simulink model "JFK_Sleep_u"  (R2015a)
settings: Solver=ode3  StartTime=0.0  StopTime=3000  FixedStep=0.01  RelTol=1e-5
values from neighbouring files (symbols this model uses):
  D = 1600/24    (= 66.6666666667)    [Periodic_Solution.m]
  H0 = 0.4    [Periodic_Solution.m]
  T = 24    [Periodic_Solution.m]
  umax = 0.1731    [Periodic_Solution.m]
  x0 = 1.06    [Periodic_Solution.m]
  xc0 = 0    [Periodic_Solution.m]
settings Model: Creator=Zhang Jiaxiang  LastModifiedBy=Jiawei Yin
settings DataIOCC: LimitDataPoints=off  SignalLoggingSaveFormat=ModelDataLogs
settings OptimizationCC: ExpressionDepthLimit=2147483647
settings DebuggingCC: UnderspecifiedInitializationDetection=Classic  MergeDetectMultiDrivingBlocksExec=none  FcnCallInpInsideContextMsg=UseLocalSettings  StateNameClashWarn=warning
settings GRTTargetCC: CombineOutputUpdateFcns=off  GRTInterface=on

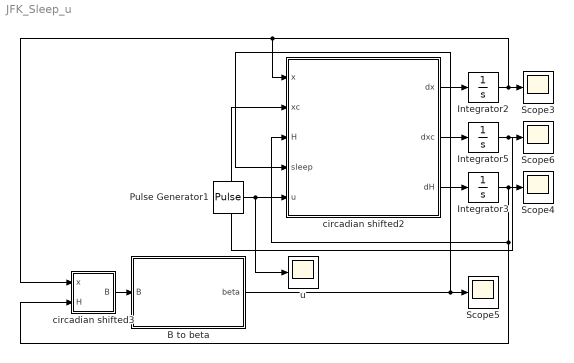
== system JFK_Sleep_u ==
  B to beta : Subsystem
  Integrator2 : Integrator  InitialCondition=x0
  Integrator3 : Integrator  InitialCondition=H0
  Integrator5 : Integrator  InitialCondition=xc0
  Pulse Generator1 : DiscretePulseGenerator  PulseType=Time based  Amplitude=umax  Period=T  PulseWidth=D
  Scope{3..6} (4 alike) : Scope
      Scope3 settings: TimeRange=auto  MaxDataPoints=5000  SaveName=x  YMin=-1.3407  YMax=1.30997  SampleTime=-1  DataFormat=Array
      Scope4 settings: TimeRange=auto  MaxDataPoints=5000  SaveName=H  YMin=0.02024  YMax=0.68165  SampleTime=-1  DataFormat=Array
      Scope5 settings: TimeRange=auto  MaxDataPoints=5000  SaveName=sleep  YMin=-0.125  YMax=1.125  SampleTime=-1  DataFormat=Array
      Scope6 settings: TimeRange=auto  MaxDataPoints=5000  SaveName=xc  YMin=-1.42896  YMax=1.30771  SampleTime=-1  DataFormat=Array
  circadian shifted2 : MATLAB Function  TreatAsAtomicUnit=on
      settings: PermitHierarchicalResolution=ParametersOnly
  circadian shifted3 : MATLAB Function  TreatAsAtomicUnit=on
      settings: PermitHierarchicalResolution=ParametersOnly
  u : Scope
      settings: TimeRange=auto  MaxDataPoints=5000  SaveName=u  YMin=-10  YMax=10  SampleTime=-1  DataFormat=Array
  wires:
  circadian shifted2/1(dx) -> Integrator2/1
  circadian shifted2/3(dH) -> Integrator3/1
  Integrator3/1 -> circadian shifted2/3(H), circadian shifted3/2(H), Scope4/1
  circadian shifted3/1(B) -> B to beta/1(B)
  B to beta/1(beta) -> Scope5/1, circadian shifted2/4(sleep)
  Integrator2/1 -> Scope3/1, circadian shifted3/1(x), circadian shifted2/1(x)
  circadian shifted2/2(dxc) -> Integrator5/1
  Integrator5/1 -> circadian shifted2/2(xc), Scope6/1
  Pulse Generator1/1 -> u/1, circadian shifted2/5(u)

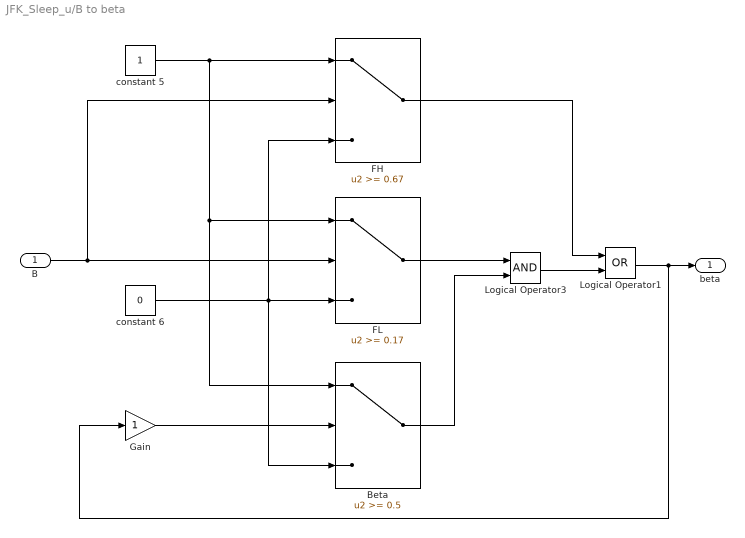
== system JFK_Sleep_u/B to beta ==
  B : Inport
  Beta : Switch  Threshold=0.5
  FH : Switch  Threshold=0.67
  FL : Switch  Threshold=0.17
  Gain : Gain
  Logical Operator1 : Logic  Operator=OR  AllPortsSameDT=off  OutDataTypeStr=boolean
  Logical Operator3 : Logic  AllPortsSameDT=off  OutDataTypeStr=boolean
  constant 5 : Constant
  constant 6 : Constant  Value=0
  beta : Outport
  wires:
  constant 5/1 -> Beta/1, FL/1, FH/1
  constant 6/1 -> Beta/3, FH/3, FL/3
  B/1 -> FH/2, FL/2
  Logical Operator1/1 -> Gain/1, beta/1
  Gain/1 -> Beta/2
  FL/1 -> Logical Operator3/1
  Beta/1 -> Logical Operator3/2
  Logical Operator3/1 -> Logical Operator1/2
  FH/1 -> Logical Operator1/1

== matlab function JFK_Sleep_u/circadian shifted2 ==
  data: x input; xc input; H input; sleep input; u input; dx output; dxc output; dH output
function [ dx,dxc,dH] = fcn(x,xc,H,sleep,u)
%#eml
q = 1/3;
taux = 24.2;
k = 0.55;
mu=0.13;

B = u*(1-0.4*x)*(1-0.4*xc)*(1-sleep);
omega0=2*pi/24.2;
tr=18.2;
td=4.2;


dx = (pi/12)*(xc + B  + mu*(1/3*x + 4/3*x^3 - 256/105*x^7));
dxc = (pi/12)*(q*B *xc - (24/(taux*0.99729))^2*x - k*B*x);
dH=(1-H)*(1-sleep)/tr-H*sleep/td;

== matlab function JFK_Sleep_u/circadian shifted3 ==
  data: x input; H input; B output
function B = fcn(x,H)
%#eml
B=H-0.1333*x;
